simulink model "awal"  (R2022b)
settings: Solver=VariableStepAuto  StartTime=0.0  StopTime=10.0  RelTol=1e-3
undefined symbols (not defined in the file or in its folder): DiscIntNeverNeededParam
libraries: simulink x8, rllib x1
settings Model: Creator=yonat  LastModifiedBy=Gesha

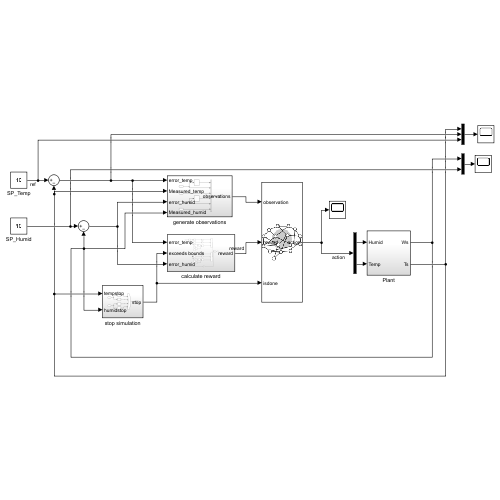
[thumbnail: Simulink's stored preview of the top-level diagram]
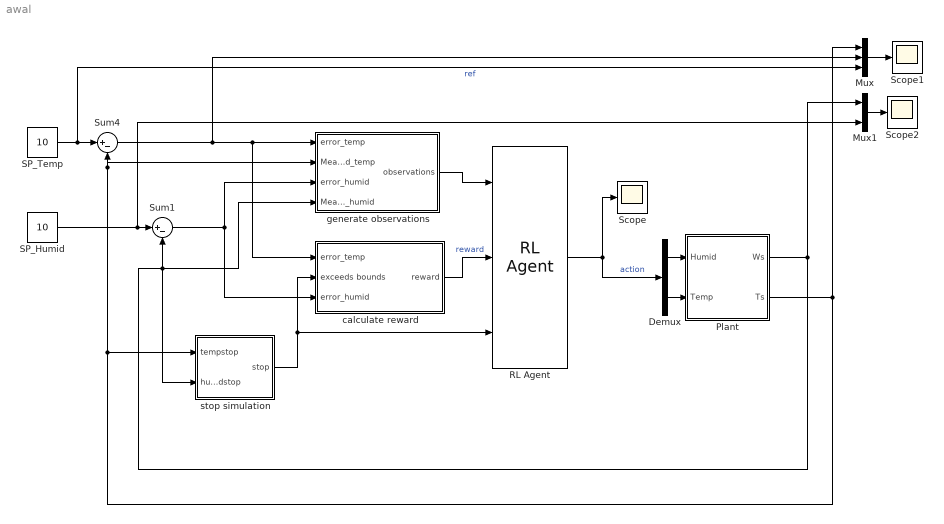
== system awal ==
  Demux : Demux  Outputs=2
  Mux : Mux  Inputs=3
  Mux1 : Mux  Inputs=2
  Plant : Subsystem
  RL Agent : rllib/RL Agent  Agent=agent  ExternalActionAsInput=off  ProvideLastAction=off  ProvideCumRwd=off  TreatAsDirectFeedthrough=on  UseStrictObservationDataTypes=off
  SP_Humid : Constant  Value=10
  SP_Temp : Constant  Value=10
  Scope : Scope
  Scope1 : Scope
  Scope2 : Scope
  Sum1 : Sum  Inputs=|+-  SaturateOnIntegerOverflow=on
  Sum4 : Sum  Inputs=|+-  SaturateOnIntegerOverflow=on
  calculate reward : Subsystem
  generate observations : Subsystem
  stop simulation : Subsystem
  wires:
  calculate reward/1(reward) -> RL Agent/2  "reward"
  stop simulation/1(stop) -> RL Agent/3, calculate reward/2(exceeds bounds)
  Sum4/1 -> Mux/2, generate observations/1(error_temp), calculate reward/1(error_temp)
  SP_Temp/1 -> Sum4/1, Mux/3  "ref"
  RL Agent/1 -> Scope/1, Demux/1  "action"
  Demux/1 -> Plant/1(Humid)
  Demux/2 -> Plant/2(Temp)
  SP_Humid/1 -> Mux1/2, Sum1/1
  Sum1/1 -> generate observations/3(error_humid), calculate reward/3(error_humid)
  Mux/1 -> Scope1/1
  Mux1/1 -> Scope2/1
  Plant/2(Ts) -> stop simulation/1(tempstop), generate observations/2(Measured_temp), Sum4/2, Mux/1
  Plant/1(Ws) -> generate observations/4(Measured_humid), stop simulation/2(humidstop), Sum1/2, Mux1/1
  generate observations/1(observations) -> RL Agent/1

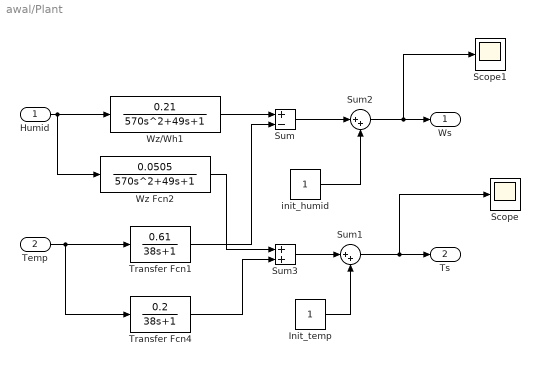
== system awal/Plant ==
  Humid : Inport
  Temp : Inport  Port=2
  Init_temp : Constant
  Scope : Scope
  Scope1 : Scope
  Sum : Sum  Inputs=+-
  Sum1 : Sum  Inputs=|++
  Sum2 : Sum  Inputs=|++
  Sum3 : Sum
  Transfer Fcn1 : TransferFcn  Numerator=[0.61]  Denominator=[38 1]
  Transfer Fcn4 : TransferFcn  Numerator=[0.2]  Denominator=[38 1]
  Wz Fcn2 : TransferFcn  Numerator=[0.0505]  Denominator=[570 49 1]
  Wz/Wh1 : TransferFcn  Numerator=[0.21]  Denominator=[570 49 1]
  init_humid : Constant
  Ws : Outport
  Ts : Outport  Port=2
  wires:
  Wz Fcn2/1 -> Sum3/1
  Humid/1 -> Wz Fcn2/1, Wz/Wh1/1
  Temp/1 -> Transfer Fcn4/1, Transfer Fcn1/1
  Transfer Fcn1/1 -> Sum/2
  Wz/Wh1/1 -> Sum/1
  Transfer Fcn4/1 -> Sum3/2
  Sum/1 -> Sum2/1
  Sum3/1 -> Sum1/1
  Sum1/1 -> Scope/1, Ts/1
  Sum2/1 -> Scope1/1, Ws/1
  Init_temp/1 -> Sum1/2
  init_humid/1 -> Sum2/2

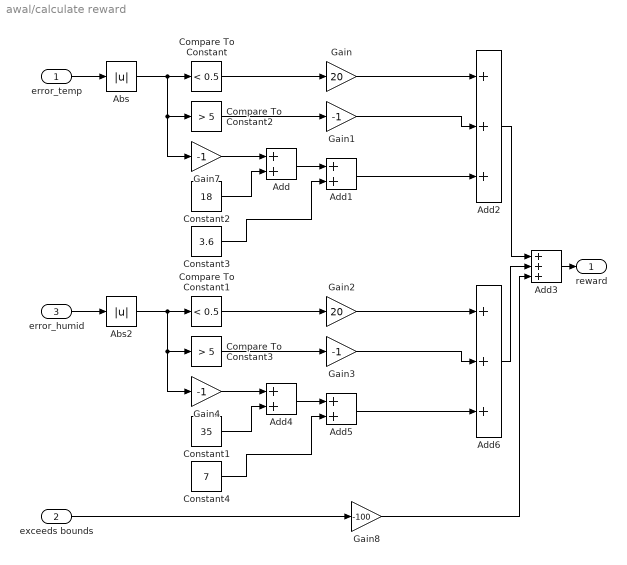
== system awal/calculate reward ==
  error_temp : Inport
  exceeds bounds : Inport  Port=2
  error_humid : Inport  Port=3
  Abs : Abs  SaturateOnIntegerOverflow=off
  Abs2 : Abs  SaturateOnIntegerOverflow=off
  Add{,1,4..5} (4 alike) : Sum
  Add2 : Sum  Inputs=+++
  Add3 : Sum  Inputs=+++
  Add6 : Sum  Inputs=+++
  Compare To Constant : simulink/Logic and Bit Operations/Compare To Constant  relop=<  const=0.5  OutDataTypeStr=boolean
  Compare To Constant1 : simulink/Logic and Bit Operations/Compare To Constant  relop=<  const=0.5  OutDataTypeStr=boolean
  Compare To Constant2 : simulink/Logic and Bit Operations/Compare To Constant  relop=>  const=5  OutDataTypeStr=boolean
  Compare To Constant3 : simulink/Logic and Bit Operations/Compare To Constant  relop=>  const=5  OutDataTypeStr=boolean
  Constant1 : Constant  Value=35
  Constant2 : Constant  Value=18
  Constant3 : Constant  Value=3.6
  Constant4 : Constant  Value=7
  Gain : Gain  Gain=20
  Gain{1,3..4,7} (4 alike) : Gain  Gain=-1
  Gain2 : Gain  Gain=20
  Gain8 : Gain  Gain=-100
  reward : Outport  VectorParamsAs1DForOutWhenUnconnected=off
  wires:
  error_temp/1 -> Abs/1
  Abs/1 -> Gain7/1, Compare To Constant2/1, Compare To Constant/1
  Compare To Constant/1 -> Gain/1
  Compare To Constant2/1 -> Gain1/1
  Gain/1 -> Add2/1
  Gain7/1 -> Add/1
  Constant2/1 -> Add/2
  Add/1 -> Add1/1
  Constant3/1 -> Add1/2
  Add1/1 -> Add2/3
  Gain1/1 -> Add2/2
  Add3/1 -> reward/1
  Add2/1 -> Add3/1
  exceeds bounds/1 -> Gain8/1
  Gain8/1 -> Add3/3
  Constant1/1 -> Add4/2
  Constant4/1 -> Add5/2
  Add4/1 -> Add5/1
  Gain2/1 -> Add6/1
  Compare To Constant3/1 -> Gain3/1
  Gain4/1 -> Add4/1
  Abs2/1 -> Gain4/1, Compare To Constant3/1, Compare To Constant1/1
  Compare To Constant1/1 -> Gain2/1
  Gain3/1 -> Add6/2
  error_humid/1 -> Abs2/1
  Add5/1 -> Add6/3
  Add6/1 -> Add3/2

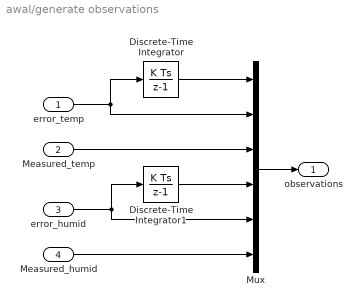
== system awal/generate observations ==
  error_temp : Inport
  Measured_temp : Inport  Port=2
  error_humid : Inport  Port=3
  Measured_humid : Inport  Port=4
  Discrete-Time Integrator : DiscreteIntegrator  SampleTime=1.0  ICPrevOutput=DiscIntNeverNeededParam  ICPrevScaledInput=DiscIntNeverNeededParam
  Discrete-Time Integrator1 : DiscreteIntegrator  SampleTime=1.0  ICPrevOutput=DiscIntNeverNeededParam  ICPrevScaledInput=DiscIntNeverNeededParam
  Mux : Mux  Inputs=6
  observations : Outport  VectorParamsAs1DForOutWhenUnconnected=off
  wires:
  error_temp/1 -> Discrete-Time Integrator/1, Mux/2
  error_humid/1 -> Mux/5, Discrete-Time Integrator1/1
  Discrete-Time Integrator1/1 -> Mux/4
  Discrete-Time Integrator/1 -> Mux/1
  Measured_temp/1 -> Mux/3
  Measured_humid/1 -> Mux/6
  Mux/1 -> observations/1

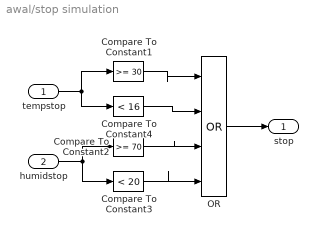
== system awal/stop simulation ==
  tempstop : Inport
  humidstop : Inport  Port=2
  Compare To Constant1 : simulink/Logic and Bit Operations/Compare To Constant  relop=>=  const=30  OutDataTypeStr=boolean
  Compare To Constant2 : simulink/Logic and Bit Operations/Compare To Constant  relop=>=  const=70  OutDataTypeStr=boolean
  Compare To Constant3 : simulink/Logic and Bit Operations/Compare To Constant  relop=<  const=20  OutDataTypeStr=boolean
  Compare To Constant4 : simulink/Logic and Bit Operations/Compare To Constant  relop=<  const=16  OutDataTypeStr=boolean
  OR : Logic  Operator=OR  Inputs=4  IconShape=distinctive  AllPortsSameDT=off  OutDataTypeStr=boolean
  stop : Outport  VectorParamsAs1DForOutWhenUnconnected=off
  wires:
  tempstop/1 -> Compare To Constant1/1, Compare To Constant4/1
  humidstop/1 -> Compare To Constant2/1, Compare To Constant3/1
  Compare To Constant2/1 -> OR/3
  Compare To Constant1/1 -> OR/1
  Compare To Constant3/1 -> OR/4
  Compare To Constant4/1 -> OR/2
  OR/1 -> stop/1
